simulink model "a_Quadrotor_Plant_Sim"  (R2018b)
settings: Solver=VariableStepAuto  StartTime=0.0  StopTime=20  RelTol=1e-3
InitFcn:
  | a_Initial
values from neighbouring files (symbols this model uses):
  B = 0.114e-06    (= 1.14e-07)    [a_Initial.m]    (also in c_Observer_Design.m = sys.b)
  g = 9.8    [a_Initial.m]
  K = 2.98e-06    [a_Initial.m]    (also in c_Observer_Design.m = place(A_Reform, B_Reform, poles))
  L = 0.225    [a_Initial.m]    (also in c_Observer_Design.m = L')
  m = 0.468    [a_Initial.m]
  X0 = [p0 q0 r0 phi0 the0 psi0 u0 v0 w0 x0 y0 z0]    [a_Initial.m]
settings Model: Creator=Milad  LastModifiedBy=Milad
settings DataIOCC: ReturnWorkspaceOutputs=on

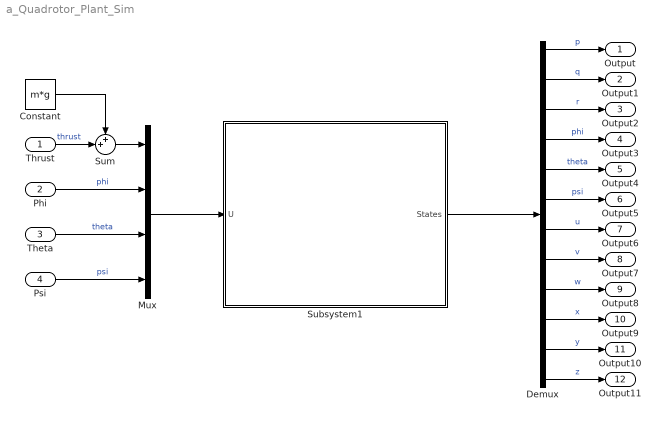
== system a_Quadrotor_Plant_Sim ==
  Thrust : Inport
  Phi : Inport  Port=2
  Theta : Inport  Port=3
  Psi : Inport  Port=4
  Constant : Constant  Value=m*g
  Demux : Demux  Outputs=12
  Mux : Mux
  Subsystem1 : Subsystem
  Sum : Sum  Inputs=++|
  Output : Outport
  Output1 : Outport  Port=2
  Output2 : Outport  Port=3
  Output3 : Outport  Port=4
  Output4 : Outport  Port=5
  Output5 : Outport  Port=6
  Output6 : Outport  Port=7
  Output7 : Outport  Port=8
  Output8 : Outport  Port=9
  Output9 : Outport  Port=10
  Output10 : Outport  Port=11
  Output11 : Outport  Port=12
  wires:
  Demux/1 -> Output/1  "p"
  Demux/2 -> Output1/1  "q"
  Demux/3 -> Output2/1  "r"
  Demux/4 -> Output3/1  "phi"
  Demux/5 -> Output4/1  "theta"
  Demux/6 -> Output5/1  "psi"
  Demux/7 -> Output6/1  "u"
  Demux/8 -> Output7/1  "v"
  Demux/9 -> Output8/1  "w"
  Demux/10 -> Output9/1  "x"
  Demux/11 -> Output10/1  "y"
  Demux/12 -> Output11/1  "z"
  Phi/1 -> Mux/2  "phi"
  Theta/1 -> Mux/3  "theta"
  Psi/1 -> Mux/4  "psi"
  Subsystem1/1(States) -> Demux/1
  Thrust/1 -> Sum/2  "thrust"
  Mux/1 -> Subsystem1/1(U)
  Sum/1 -> Mux/1
  Constant/1 -> Sum/1

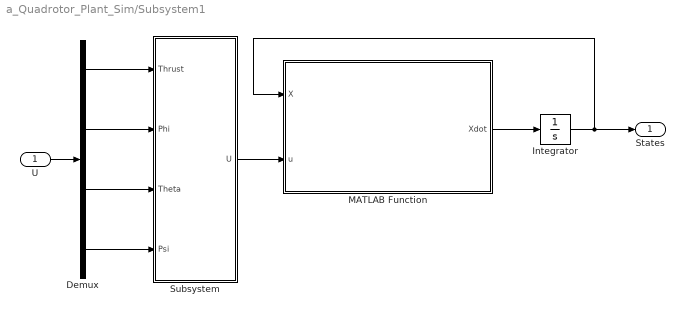
== system a_Quadrotor_Plant_Sim/Subsystem1 ==
  U : Inport
  Demux : Demux
  Integrator : Integrator  InitialCondition=X0
  MATLAB Function : MATLAB Function  TreatAsAtomicUnit=on
  Subsystem : Subsystem
  States : Outport
  wires:
  Demux/4 -> Subsystem/4(Psi)
  Demux/2 -> Subsystem/2(Phi)
  Subsystem/1(U) -> MATLAB Function/2(u)
  Integrator/1 -> States/1, MATLAB Function/1(X)
  Demux/1 -> Subsystem/1(Thrust)
  MATLAB Function/1(Xdot) -> Integrator/1
  Demux/3 -> Subsystem/3(Theta)
  U/1 -> Demux/1

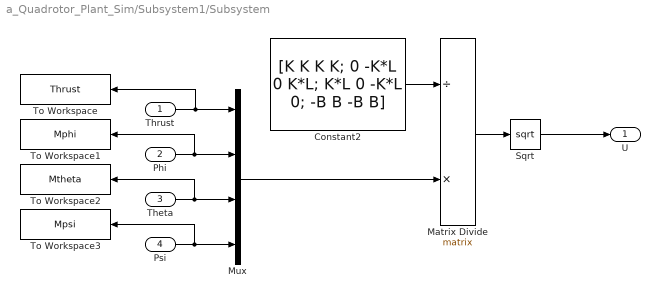
== system a_Quadrotor_Plant_Sim/Subsystem1/Subsystem ==
  Thrust : Inport
  Phi : Inport  Port=2
  Theta : Inport  Port=3
  Psi : Inport  Port=4
  Constant2 : Constant  Value=[K K K K; 0 -K*L 0 K*L; K*L 0 -K*L 0; -B B -B B]
  Matrix Divide : Product  Inputs=/*  Multiplication=Matrix(*)
  Mux : Mux
  Sqrt : Sqrt  SaturateOnIntegerOverflow=on
  To Workspace : ToWorkspace  VariableName=Thrust  SampleTime=-1
  To Workspace1 : ToWorkspace  VariableName=Mphi  SampleTime=-1
  To Workspace2 : ToWorkspace  VariableName=Mtheta  SampleTime=-1
  To Workspace3 : ToWorkspace  VariableName=Mpsi  SampleTime=-1
  U : Outport
  wires:
  Matrix Divide/1 -> Sqrt/1
  Thrust/1 -> To Workspace/1, Mux/1
  Psi/1 -> To Workspace3/1, Mux/4
  Phi/1 -> To Workspace1/1, Mux/2
  Mux/1 -> Matrix Divide/2
  Constant2/1 -> Matrix Divide/1
  Theta/1 -> To Workspace2/1, Mux/3
  Sqrt/1 -> U/1

== matlab function a_Quadrotor_Plant_Sim/Subsystem1/MATLAB Function ==
  data: X input; Xdot output; u input
function Xdot = Quadrotor_Model(X, u)

k   = 2.98e-06;
b   = 0.114e-06;
d   = b/k;
l   = 0.225;
m   = 0.468;
Ixx = 4.856e-03;
Iyy = 4.856e-03;
Izz = 8.801e-03;
Ir  = 3.357e-05;
Ax  = 0.3;
Ay  = 0.3;
Az  = 0.25;
Ar  = 0.2;
g   = 9.8;

P = X(1);
Q = X(2);
R = X(3);

Phi = X(4);
The = X(5);
Psi = X(6);

U = X(7);
V = X(8);
W = X(9);

x = X(10);
Y = X(11);
Z = X(12);

w1 = u(1);
w2 = u(2);
w3 = u(3);
w4 = u(4);

T1= k*w1^2;
T2= k*w2^2;
T3= k*w3^2;
T4= k*w4^2;

T    = T1+T2+T3+T4;
Mphi = l*(T4-T2);
Mthe = l*(T3-T1);
Mpsi = d*(-T1+T2-T3+T4);

Omega = w1-w2+w3-w4;

dP = ((Iyy-Izz)/Ixx)*Q*R - Ir/Ixx * Q*Omega + Mphi/Ixx - Ar/Ixx*P;
dQ = ((Izz-Ixx)/Iyy)*P*R + Ir/Iyy * P*Omega + Mthe/Iyy - Ar/Iyy*Q;
dR = ((Ixx-Iyy)/Izz)*P*Q + Mpsi/Izz -Ar/Izz*R;

dPhi   = P+ sin(Phi)*tan(The)*Q + cos(Phi)*tan(The)*R;
dTheta = cos(Phi)*Q - sin(Phi)*R;
dPsi   = sin(Phi)/cos(The)*Q + cos(Phi)/cos(The)*R;

dU = ( sin(Phi)*sin(Psi) + cos(Phi)*sin(The)*cos(Psi) )*T/m - Ax/m*U;
dV = ( -sin(Phi)*cos(Psi) + cos(Phi)*sin(The)*sin(Psi) )*T/m - Ay/m*V;
dW = -g + cos(Phi)*cos(The)*T/m - Az/m*W;

dX = U;
dY = V;
dZ = W;

Xdot = [dP dQ dR dPhi dTheta dPsi dU dV dW dX dY dZ]';
